simulink model "edf_semiThrottled"  (R2020a)
settings: Solver=FixedStepDiscrete  StartTime=0.0  StopTime=10.0  FixedStep=0.01  RelTol=1e-3
settings Model: OrderedModelArguments=off  Creator=developer  LastModifiedBy=developer
settings OptimizationCC: DefaultParameterBehavior=Inlined  EnhancedBackFolding=on  EnableMemcpy=off  PassReuseOutputArgsAs=Individual arguments  ZeroExternalMemoryAtStartup=off  ZeroInternalMemoryAtStartup=off  InitFltsAndDblsToZero=on  OptimizeBlockOrder=speed  DifferentSizesBufferReuse=on  EfficientTunableParamExpr=on
settings DebuggingCC: ParameterTunabilityLossMsg=error
settings SFSimCC: MATLABDynamicMemAlloc=off
settings RTWCC: SystemTargetFile=ert.tlc  GenCodeOnly=on  TemplateMakefile=ert_default_tmf
settings CodeAppCC: ForceParamTrailComments=on  IgnoreCustomStorageClasses=off  OperatorAnnotations=on  SimulinkDataObjDesc=on  SFDataObjDesc=on  InsertBlockDesc=on
settings ERTTargetCC: TargetLangStandard=C99 (ISO)  SupportNonFinite=off  SupportComplex=off  InlinedParameterPlacement=NonHierarchical  ERTCustomFileTemplate=example_file_process.tlc

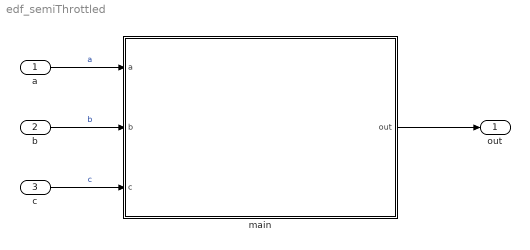
== system edf_semiThrottled ==
  a : Inport
  b : Inport  Port=2
  c : Inport  Port=3
  main : Subsystem  TreatAsAtomicUnit=on
      settings: RTWSystemCode=Nonreusable function
  out : Outport
  wires:
  a/1 -> main/1(a)  "a"
  b/1 -> main/2(b)  "b"
  c/1 -> main/3(c)  "c"
  main/1(out) -> out/1

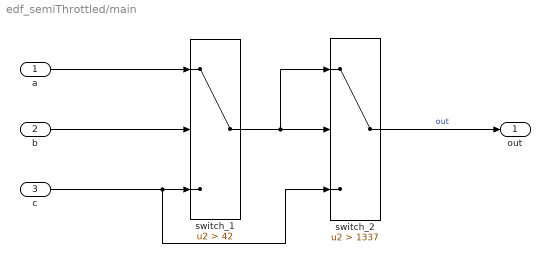
== system edf_semiThrottled/main ==
  a : Inport
  b : Inport  Port=2
  c : Inport  Port=3
  switch_1 : Switch  Criteria=u2 > Threshold  Threshold=42
  switch_2 : Switch  Criteria=u2 > Threshold  Threshold=1337
  out : Outport
  wires:
  c/1 -> switch_2/3, switch_1/3
  switch_1/1 -> switch_2/1, switch_2/2
  a/1 -> switch_1/1
  b/1 -> switch_1/2
  switch_2/1 -> out/1  "out"
